simulink model "trial"  (R2021b)
settings: Solver=FixedStepAuto  StartTime=0.0  StopTime=inf  FixedStep=0.01  RelTol=1e-3
libraries: robotlib x1
settings Model: Creator=Asus ROG  LastModifiedBy=Asus ROG

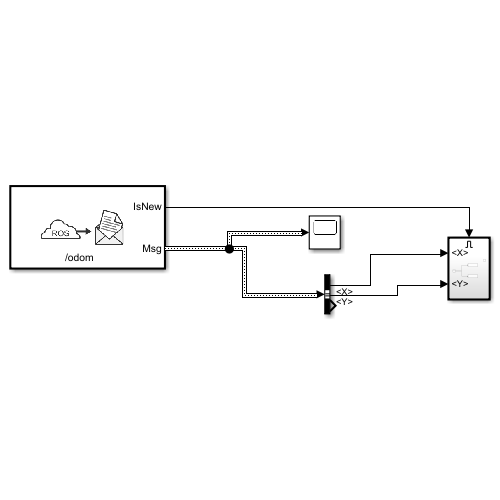
[thumbnail: Simulink's stored preview of the top-level diagram]
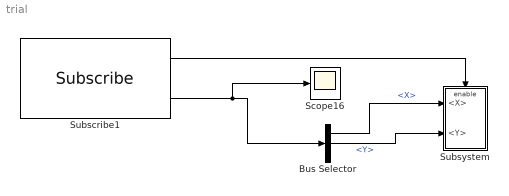
== system trial ==
  Bus Selector : BusSelector  OutputSignals=Pose.Pose.Position.X,Pose.Pose.Position.Y,Pose.Pose.Orientation.Z
  Scope16 : Scope
  Subscribe1 : robotlib/Subscribe  topicSource=Select from ROS network  topic=/odom  messageType=nav_msgs/Odometry  SampleTime=-1  legacyBusStruct=off  messageQueueLength=1
  Subsystem : Subsystem
  wires:
  Subscribe1/2 -> Scope16/1, Bus Selector/1
  Bus Selector/1 -> Subsystem/1(<X>)  "<X>"
  Bus Selector/2 -> Subsystem/2(<Y>)  "<Y>"
  Subscribe1/1 -> Subsystem/Enable

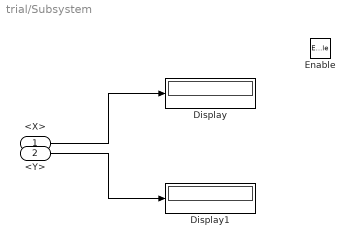
== system trial/Subsystem ==
  <X> : Inport
  <Y> : Inport  Port=2
  Enable : EnablePort
  Display : Display
  Display1 : Display
  wires:
  <Y>/1 -> Display1/1
  <X>/1 -> Display/1
